simulink model "EHB_speedgoat_R2020a_V1"  (R2020a)
settings: Solver=FixedStepDiscrete  StartTime=0.0  StopTime=inf  FixedStep=0.001  RelTol=1e-3  EnableMultiTasking=on
model workspace (MAT data in the model file):
  A : Simulink.Signal (value not decoded)
  B : Simulink.Signal (value not decoded)
  C : Simulink.Signal (value not decoded)
  D : Simulink.Signal (value not decoded)
  E : Simulink.Signal (value not decoded)
  calin = [-9.96 -7.98 -5.98 -3.99 -1.994 0 1.995 3.992 5.99 7.98 9.97]
  calout = [-10 -8 -6 -4 -2 0 2 4 6 8 10]
symbols that are objects in the model workspace (value not decoded): C, D
undefined symbols (not defined in the file): Com1, none, ts_IO612
libraries: simulink x1436, xpcethercatlib x1223, yisutbxlib_utilities x256, xpcutilitieslib x156, hdlsllib x145, canmsglib x46, speedgoatlib_IO602_4 x11, speedgoatlib_IO611 x7, slrttcplib x4, CanManageLib x3, slrtlib x3, xpcseriallib x2
(part 7 of 30)

== system EHB_speedgoat_R2020a_V1/保留/TIF_02/CB3012_01/Res2Cmd6 ==
  ResVal : Inport
  Add : Sum  Inputs=-+
  Constant : Constant
  Divide : Product  Inputs=*/  OutDataTypeStr=uint16  RndMeth=Round
  MaxResVal : Constant  Value=1e6  OutDataTypeStr=Inherit: Inherit via back propagation
  Switch : Switch  Criteria=u2 > Threshold  OutDataTypeStr=Inherit: Inherit via back propagation
  zero : Constant  Value=0  OutDataTypeStr=Inherit: Inherit via back propagation
  CmdVal : Outport
  wires:
  MaxResVal/1 -> Divide/1
  Divide/1 -> Switch/1
  Switch/1 -> CmdVal/1
  zero/1 -> Switch/3
  ResVal/1 -> Add/2
  Add/1 -> Divide/2, Switch/2
  Constant/1 -> Add/1

== system EHB_speedgoat_R2020a_V1/保留/TIF_02/CB3012_01/Res2Cmd7 ==
  ResVal : Inport
  Add : Sum  Inputs=-+
  Constant : Constant
  Divide : Product  Inputs=*/  OutDataTypeStr=uint16  RndMeth=Round
  MaxResVal : Constant  Value=1e6  OutDataTypeStr=Inherit: Inherit via back propagation
  Switch : Switch  Criteria=u2 > Threshold  OutDataTypeStr=Inherit: Inherit via back propagation
  zero : Constant  Value=0  OutDataTypeStr=Inherit: Inherit via back propagation
  CmdVal : Outport
  wires:
  Constant/1 -> Add/1
  Add/1 -> Switch/2, Divide/2
  ResVal/1 -> Add/2
  zero/1 -> Switch/3
  Switch/1 -> CmdVal/1
  Divide/1 -> Switch/1
  MaxResVal/1 -> Divide/1

== system EHB_speedgoat_R2020a_V1/保留/TIF_02/CB3012_01/Res2Cmd8 ==
  ResVal : Inport
  Add : Sum  Inputs=-+
  Constant : Constant
  Divide : Product  Inputs=*/  OutDataTypeStr=uint16  RndMeth=Round
  MaxResVal : Constant  Value=1e6  OutDataTypeStr=Inherit: Inherit via back propagation
  Switch : Switch  Criteria=u2 > Threshold  OutDataTypeStr=Inherit: Inherit via back propagation
  zero : Constant  Value=0  OutDataTypeStr=Inherit: Inherit via back propagation
  CmdVal : Outport
  wires:
  MaxResVal/1 -> Divide/1
  Divide/1 -> Switch/1
  Switch/1 -> CmdVal/1
  zero/1 -> Switch/3
  ResVal/1 -> Add/2
  Add/1 -> Divide/2, Switch/2
  Constant/1 -> Add/1

== system EHB_speedgoat_R2020a_V1/保留/TIF_02/CB3012_01/Res2Cmd9 ==
  ResVal : Inport
  Add : Sum  Inputs=-+
  Constant : Constant
  Divide : Product  Inputs=*/  OutDataTypeStr=uint16  RndMeth=Round
  MaxResVal : Constant  Value=1e6  OutDataTypeStr=Inherit: Inherit via back propagation
  Switch : Switch  Criteria=u2 > Threshold  OutDataTypeStr=Inherit: Inherit via back propagation
  zero : Constant  Value=0  OutDataTypeStr=Inherit: Inherit via back propagation
  CmdVal : Outport
  wires:
  Constant/1 -> Add/1
  Add/1 -> Switch/2, Divide/2
  ResVal/1 -> Add/2
  zero/1 -> Switch/3
  Switch/1 -> CmdVal/1
  Divide/1 -> Switch/1
  MaxResVal/1 -> Divide/1

== system EHB_speedgoat_R2020a_V1/保留/TIF_03/CB1032_3/DIO ==
  DI : Subsystem  mask(simucat_di){deviceID=0, boxNum=Box 3 (Digital Board), channel1=on, channel2=on, channel3=on, channel4=on, channel5=on, channel6=on, channel7=on, channel8=on, channel9=on, channel10=on, channel11=on, channel12=on, channel13=on, channel14=on, channel15=on, channel16=on, channel17=on, channel18=on, channel19=on, channel20=on, channel21=on, channel22=on, channel23=on, channel24=on, channel25=on, channel26=on, channel27=on, channel28=on, channel29=on, channel30=on, channel31=on, channel32=on}
      mask prompts: deviceID "Device Index:"; boxNum "Select a box:"; channel1 "1"; channel2 "2"; channel3 "3"; channel4 "4"; channel5 "5"; channel6 "6"; channel7 "7"; channel8 "8"; channel9 "9"; channel10 "10"; channel11 "11"; channel12 "12"; channel13 "13"; channel14 "14"; channel15 "15"; channel16 "16"; channel17 "17"; channel18 "18"; channel19 "19"; channel20 "20"; channel21 "21"; channel22 "22"; channel23 "23"; channel24 "24"; channel25 "25"; channel26 "26"; channel27 "27"; channel28 "28"; channel29 "29"; channel30 "30"; channel31 "31"; channel32 "32"
      mask help:
      | SimuCat系列数字板卡驱动模块。
      | 功能：数字量输入。通道数：32
      mask TypeOptions deviceID: 0 | 1 | 2 | 3 | 4 | 5 | 6 | 7 | 8 | 9 | 10 | 11 | 12 | 13 | 14 | 15
      mask TypeOptions boxNum: Box 1 (Digital Board) | Box 2 (Digital Board) | Box 3 (Digital Board) | Box 4 (Digital Board)
      mask DialogControl refreshButton Prompt: Refresh
      mask DialogControl refreshButton Callback: ystbx.mask.callbacks.refreshBoxList
      mask DialogControl selectChannel Prompt: Select channels:
      mask DialogControl Dummy Prompt: (Add text here)
      mask DialogControl channelSelectAll Prompt: Select All
      mask DialogControl channelSelectAll Callback: ystbx.mask.callbacks.selectAllChannels();
      mask DialogControl channelClearAll Prompt: Clear All
      mask DialogControl channelClearAll Callback: ystbx.mask.callbacks.clearAllChannels();
      mask DialogControl applyButton Prompt: Apply Modification
      mask DialogControl applyButton Callback: ystbx.mask.callbacks.maskApply();
      mask Display: disp('CB1032(Digital Board)\ndigital signal input\nNetwork Device 0\nBox 3 (Digital Board)');port_label('output',1,'DI_CH1');port_label('output',2,'DI_CH2');port_label('output',3,'DI_CH3');port_label('output',4,'DI_CH4');port_label('output',5,'DI_CH5');port_label('output',6,'DI_CH6');port_label('output',7,'DI_CH7');port_label('output',8,'DI_CH8');port_label('output',9,'DI_CH9');port_label('output',10,'DI_CH10');port_label('output',11,'DI_CH11');port_label('output',12,'DI_CH12');port_label('output',13,'DI_CH13');port_label('output',14,'DI_CH14');port_label('output',15,'DI_CH15');port_label('output',16,'DI_CH16');port_label('output',17,'DI_CH17');port_label('output',18,'DI_CH18');port_label('output',19,'DI_CH19');port_label('output',20,'DI_CH20');port_label('output',21,'DI_CH21');port_label('output',22,'DI_CH22');port_label('output',23,'DI_CH23');port_label('output',24,'DI_CH24');port_label('output',25,'DI_CH25');port_label('output',26,'DI_CH26');port_label('output',27,'DI_CH27');port_label('output',28,'DI_CH28');port_label('output',29,'DI_CH29');port_label('output',30,'DI_CH30');port_label('output',31,'DI_CH31');port_label('output',32,'DI_CH32');
  DI_{1..32} (32 alike) : Gain  OutDataTypeStr=Inherit: Inherit via back propagation
  DO : Subsystem  mask(simucat_do){deviceID=0, boxNum=Box 3 (Digital Board), channel1=on, channel2=on, channel3=on, channel4=on, channel5=on, channel6=on, channel7=on, channel8=on, channel9=on, channel10=on, channel11=on, channel12=on, channel13=on, channel14=on, channel15=on, channel16=on, channel17=on, channel18=on, channel19=on, channel20=on, channel21=on, channel22=on, channel23=on, channel24=on, channel25=on, channel26=on, channel27=on, channel28=on, channel29=on, channel30=on, channel31=on, channel32=on, enableSetMode=off}
      mask prompts: deviceID "Device Index:"; boxNum "Select a box:"; channel1 "1"; channel2 "2"; channel3 "3"; channel4 "4"; channel5 "5"; channel6 "6"; channel7 "7"; channel8 "8"; channel9 "9"; channel10 "10"; channel11 "11"; channel12 "12"; channel13 "13"; channel14 "14"; channel15 "15"; channel16 "16"; channel17 "17"; channel18 "18"; channel19 "19"; channel20 "20"; channel21 "21"; channel22 "22"; channel23 "23"; channel24 "24"; channel25 "25"; channel26 "26"; channel27 "27"; channel28 "28"; channel29 "29"; channel30 "30"; channel31 "31"; channel32 "32"; enableSetMode "Enable SetMode"
      mask help:
      | SimuCat系列数字板卡驱动模块。
      | 功能：数字量输出。通道数：32
      mask TypeOptions deviceID: 0 | 1 | 2 | 3 | 4 | 5 | 6 | 7 | 8 | 9 | 10 | 11 | 12 | 13 | 14 | 15
      mask TypeOptions boxNum: Box 1 (Digital Board) | Box 2 (Digital Board) | Box 3 (Digital Board) | Box 4 (Digital Board)
      mask DialogControl refreshButton Prompt: Refresh
      mask DialogControl refreshButton Callback: ystbx.mask.callbacks.refreshBoxList
      mask DialogControl selectChannel Prompt: Select channels:
      mask DialogControl Dummy Prompt: (Add text here)
      mask DialogControl channelSelectAll Prompt: Select All
      mask DialogControl channelSelectAll Callback: ystbx.mask.callbacks.selectAllChannels();
      mask DialogControl channelClearAll Prompt: Clear All
      mask DialogControl channelClearAll Callback: ystbx.mask.callbacks.clearAllChannels();
      mask DialogControl applyButton Prompt: Apply Modification
      mask DialogControl applyButton Callback: ystbx.mask.callbacks.maskApply();
      mask Display: disp('CB1032(Digital Board)\ndigital signal output\nNetwork Device 0\nBox 3 (Digital Board)');port_label('input',1,'DO_CH1');port_label('input',2,'DO_CH2');port_label('input',3,'DO_CH3');port_label('input',4,'DO_CH4');port_label('input',5,'DO_CH5');port_label('input',6,'DO_CH6');port_label('input',7,'DO_CH7');port_label('input',8,'DO_CH8');port_label('input',9,'DO_CH9');port_label('input',10,'DO_CH10');port_label('input',11,'DO_CH11');port_label('input',12,'DO_CH12');port_label('input',13,'DO_CH13');port_label('input',14,'DO_CH14');port_label('input',15,'DO_CH15');port_label('input',16,'DO_CH16');port_label('input',17,'DO_CH17');port_label('input',18,'DO_CH18');port_label('input',19,'DO_CH19');port_label('input',20,'DO_CH20');port_label('input',21,'DO_CH21');port_label('input',22,'DO_CH22');port_label('input',23,'DO_CH23');port_label('input',24,'DO_CH24');port_label('input',25,'DO_CH25');port_label('input',26,'DO_CH26');port_label('input',27,'DO_CH27');port_label('input',28,'DO_CH28');port_label('input',29,'DO_CH29');port_label('input',30,'DO_CH30');port_label('input',31,'DO_CH31');port_label('input',32,'DO_CH32');
  DO_{1..32} (32 alike) : Constant  Value=0  OutDataTypeStr=Inherit: Inherit via back propagation
  Display{64..95} (32 alike) : Display
  wires:
  DI_28/1 -> Display85/1  "DI_28"
  DI_20/1 -> Display75/1  "DI_20"
  DI_7/1 -> Display68/1  "DI_7"
  DI_26/1 -> Display84/1  "DI_26"
  DI_12/1 -> Display81/1  "DI_12"
  DI_4/1 -> Display65/1  "DI_4"
  DI_18/1 -> Display82/1  "DI_18"
  DI_22/1 -> Display77/1  "DI_22"
  DI_25/1 -> Display80/1  "DI_25"
  DI_8/1 -> Display69/1  "DI_8"
  DI_11/1 -> Display72/1  "DI_11"
  DI_9/1 -> Display70/1  "DI_9"
  DI_1/1 -> Display64/1  "DI_1"
  DI_15/1 -> Display92/1  "DI_15"
  DI_3/1 -> Display95/1  "DI_3"
  DI_10/1 -> Display73/1  "DI_10"
  DI_5/1 -> Display66/1  "DI_5"
  DI_16/1 -> Display94/1  "DI_16"
  DI_2/1 -> Display71/1  "DI_2"
  DI_17/1 -> Display74/1  "DI_17"
  DI_14/1 -> Display91/1  "DI_14"
  DI_6/1 -> Display67/1  "DI_6"
  DI_13/1 -> Display93/1  "DI_13"
  DI_29/1 -> Display88/1  "DI_29"
  DI_19/1 -> Display90/1  "DI_19"
  DI_24/1 -> Display79/1  "DI_24"
  DI_30/1 -> Display86/1  "DI_30"
  DI_32/1 -> Display89/1  "DI_32"
  DI_27/1 -> Display83/1  "DI_27"
  DI_23/1 -> Display78/1  "DI_23"
  DI_31/1 -> Display87/1  "DI_31"
  DI_21/1 -> Display76/1  "DI_21"
  DO_1/1 -> DO/1(DO_CH1)  "DO_1"
  DO_2/1 -> DO/2(DO_CH2)  "DO_2"
  DO_3/1 -> DO/3(DO_CH3)  "DO_3"
  DO_4/1 -> DO/4(DO_CH4)  "DO_4"
  DO_5/1 -> DO/5(DO_CH5)  "DO_5"
  DO_6/1 -> DO/6(DO_CH6)  "DO_6"
  DO_7/1 -> DO/7(DO_CH7)  "DO_7"
  DO_8/1 -> DO/8(DO_CH8)  "DO_8"
  DO_9/1 -> DO/9(DO_CH9)  "DO_9"
  DO_10/1 -> DO/10(DO_CH10)  "DO_10"
  DO_11/1 -> DO/11(DO_CH11)  "DO_11"
  DO_12/1 -> DO/12(DO_CH12)  "DO_12"
  DO_13/1 -> DO/13(DO_CH13)  "DO_13"
  DO_14/1 -> DO/14(DO_CH14)  "DO_14"
  DO_15/1 -> DO/15(DO_CH15)  "DO_15"
  DO_16/1 -> DO/16(DO_CH16)  "DO_16"
  DO_17/1 -> DO/17(DO_CH17)  "DO_17"
  DO_18/1 -> DO/18(DO_CH18)  "DO_18"
  DO_19/1 -> DO/19(DO_CH19)  "DO_19"
  DO_20/1 -> DO/20(DO_CH20)  "DO_20"
  DO_21/1 -> DO/21(DO_CH21)  "DO_21"
  DO_22/1 -> DO/22(DO_CH22)  "DO_22"
  DO_23/1 -> DO/23(DO_CH23)  "DO_23"
  DO_24/1 -> DO/24(DO_CH24)  "DO_24"
  DO_25/1 -> DO/25(DO_CH25)  "DO_25"
  DO_26/1 -> DO/26(DO_CH26)  "DO_26"
  DO_27/1 -> DO/27(DO_CH27)  "DO_27"
  DO_28/1 -> DO/28(DO_CH28)  "DO_28"
  DO_29/1 -> DO/29(DO_CH29)  "DO_29"
  DO_30/1 -> DO/30(DO_CH30)  "DO_30"
  DO_31/1 -> DO/31(DO_CH31)  "DO_31"
  DO_32/1 -> DO/32(DO_CH32)  "DO_32"
  DI/1(DI_CH1) -> DI_1/1
  DI/2(DI_CH2) -> DI_2/1
  DI/3(DI_CH3) -> DI_3/1
  DI/4(DI_CH4) -> DI_4/1
  DI/5(DI_CH5) -> DI_5/1
  DI/6(DI_CH6) -> DI_6/1
  DI/7(DI_CH7) -> DI_7/1
  DI/8(DI_CH8) -> DI_8/1
  DI/9(DI_CH9) -> DI_9/1
  DI/10(DI_CH10) -> DI_10/1
  DI/11(DI_CH11) -> DI_11/1
  DI/12(DI_CH12) -> DI_12/1
  DI/13(DI_CH13) -> DI_13/1
  DI/14(DI_CH14) -> DI_14/1
  DI/15(DI_CH15) -> DI_15/1
  DI/16(DI_CH16) -> DI_16/1
  DI/17(DI_CH17) -> DI_17/1
  DI/18(DI_CH18) -> DI_18/1
  DI/19(DI_CH19) -> DI_19/1
  DI/20(DI_CH20) -> DI_20/1
  DI/21(DI_CH21) -> DI_21/1
  DI/22(DI_CH22) -> DI_22/1
  DI/23(DI_CH23) -> DI_23/1
  DI/24(DI_CH24) -> DI_24/1
  DI/25(DI_CH25) -> DI_25/1
  DI/26(DI_CH26) -> DI_26/1
  DI/27(DI_CH27) -> DI_27/1
  DI/28(DI_CH28) -> DI_28/1
  DI/29(DI_CH29) -> DI_29/1
  DI/30(DI_CH30) -> DI_30/1
  DI/31(DI_CH31) -> DI_31/1
  DI/32(DI_CH32) -> DI_32/1

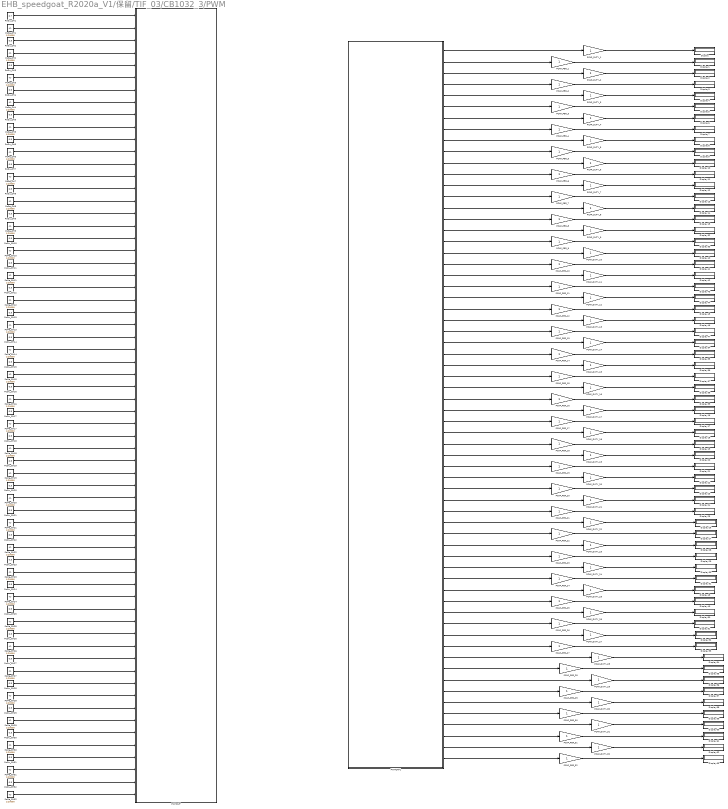
== system EHB_speedgoat_R2020a_V1/保留/TIF_03/CB1032_3/PWM ==
  Display{,1..63} (64 alike) : Display
  PCAP_DUTY_{1..32} (32 alike) : Gain
  PCAP_PER_{1..32} (32 alike) : Gain
  PWMCAP1 : Subsystem  mask(simucat_pwmcap){deviceID=0, boxNum=Box 3 (Digital Board), channel1=on, channel2=on, channel3=on, channel4=on, channel5=on, channel6=on, channel7=on, channel8=on, channel9=on, channel10=on, channel11=on, channel12=on, channel13=on, channel14=on, channel15=on, channel16=on, channel17=on, channel18=on, channel19=on, channel20=on, channel21=on, channel22=on, channel23=on, channel24=on, channel25=on, channel26=on, channel27=on, channel28=on, channel29=on, channel30=on, channel31=on, channel32=on, capMode=automatic}
      mask prompts: deviceID "Device Index:"; boxNum "Select a box:"; channel1 "1"; channel2 "2"; channel3 "3"; channel4 "4"; channel5 "5"; channel6 "6"; channel7 "7"; channel8 "8"; channel9 "9"; channel10 "10"; channel11 "11"; channel12 "12"; channel13 "13"; channel14 "14"; channel15 "15"; channel16 "16"; channel17 "17"; channel18 "18"; channel19 "19"; channel20 "20"; channel21 "21"; channel22 "22"; channel23 "23"; channel24 "24"; channel25 "25"; channel26 "26"; channel27 "27"; channel28 "28"; channel29 "29"; channel30 "30"; channel31 "31"; channel32 "32"; capMode "Cap Mode"
      mask help:
      | SimuCat系列数字板卡驱动模块。
      | 功能：PWM波捕获。通道数：32
      mask TypeOptions deviceID: 0 | 1 | 2 | 3 | 4 | 5 | 6 | 7 | 8 | 9 | 10 | 11 | 12 | 13 | 14 | 15
      mask TypeOptions boxNum: Box 1 (Digital Board) | Box 2 (Digital Board) | Box 3 (Digital Board) | Box 4 (Digital Board)
      mask TypeOptions capMode: automatic | manual
      mask DialogControl refreshButton Prompt: Refresh
      mask DialogControl refreshButton Callback: ystbx.mask.callbacks.refreshBoxList
      mask DialogControl selectChannel Prompt: Select channels:
      mask DialogControl Dummy Prompt: (Add text here)
      mask DialogControl channelSelectAll Prompt: Select All
      mask DialogControl channelSelectAll Callback: ystbx.mask.callbacks.selectAllChannels();
      mask DialogControl channelClearAll Prompt: Clear All
      mask DialogControl channelClearAll Callback: ystbx.mask.callbacks.clearAllChannels();
      mask DialogControl applyButton Prompt: Apply Modification
      mask DialogControl applyButton Callback: ystbx.mask.callbacks.maskApply();
      mask Display: disp('CB1032(Digital Board)\nPWM signal capture\nNetwork Device 0\nBox 3 (Digital Board)');port_label('output',1,'PWMCAP_DutyCycle_CH1');port_label('output',2,'PWMCAP_Period_CH1');port_label('output',3,'PWMCAP_DutyCycle_CH2');port_label('output',4,'PWMCAP_Period_CH2');port_label('output',5,'PWMCAP_DutyCycle_CH3');port_label('output',6,'PWMCAP_Period_CH3');port_label('output',7,'PWMCAP_DutyCycle_CH4');port_label('output',8,'PWMCAP_Period_CH4');port_label('output',9,'PWMCAP_DutyCycle_CH5');port_label('output',10,'PWMCAP_Period_CH5');port_label('output',11,'PWMCAP_DutyCycle_CH6');port_label('output',12,'PWMCAP_Period_CH6');port_label('output',13,'PWMCAP_DutyCycle_CH7');port_label('output',14,'PWMCAP_Period_CH7');port_label('output',15,'PWMCAP_DutyCycle_CH8');port_label('output',16,'PWMCAP_Period_CH8');port_label('output',17,'PWMCAP_DutyCycle_CH9');port_label('output',18,'PWMCAP_Period_CH9');port_label('output',19,'PWMCAP_DutyCycle_CH10');port_label('output',20,'PWMCAP_Period_CH10');port_label('output',21,'PWMCAP_DutyCycle_CH11');port_label('output',22,'PWMCAP_Period_CH11');port_label('output',23,'PWMCAP_DutyCycle_CH12');port_label('output',24,'PWMCAP_Period_CH12');port_label('output',25,'PWMCAP_DutyCycle_CH13');port_label('output',26,'PWMCAP_Period_CH13');port_label('output',27,'PWMCAP_DutyCycle_CH14');port_label('output',28,'PWMCAP_Period_CH14');port_label('output',29,'PWMCAP_DutyCycle_CH15');port_label('output',30,'PWMCAP_Period_CH15');port_label('output',31,'PWMCAP_DutyCycle_CH16');port_label('output',32,'PWMCAP_Period_CH16');port_label('output',33,'PWMCAP_DutyCycle_CH17');port_label('output',34,'PWMCAP_Period_CH17');port_label('output',35,'PWMCAP_DutyCycle_CH18');port_label('output',36,'PWMCAP_Period_CH18');port_label('output',37,'PWMCAP_DutyCycle_CH19');port_label('output',38,'PWMCAP_Period_CH19');port_label('output',39,'PWMCAP_DutyCycle_CH20');port_label('output',40,'PWMCAP_Period_CH20');port_label('output',41,'PWMCAP_DutyCycle_CH21');port_label('output',42,'PWMCAP_Period_CH21');port_label('output',43,'PWMCAP_DutyCycle_CH22');port_label('output',44,'PWMCAP_Period_CH22');port_label('output',45,'PWMCAP_DutyCycle_CH23');port_label('output',46,'PWMCAP_Period_CH23');port_label('output',47,'PWMCAP_DutyCycle_CH24');port_label('output',48,'PWMCAP_Period_CH24');port_label('output',49,'PWMCAP_DutyCycle_CH25');port_label('output',50,'PWMCAP_Period_CH25');port_label('output',51,'PWMCAP_DutyCycle_CH26');port_label('output',52,'PWMCAP_Period_CH26');port_label('output',53,'PWMCAP_DutyCycle_CH27');port_label('output',54,'PWMCAP_Period_CH27');port_label('output',55,'PWMCAP_DutyCycle_CH28');port_label('output',56,'PWMCAP_Period_CH28');port_label('output',57,'PWMCAP_DutyCycle_CH29');port_label('output',58,'PWMCAP_Period_CH29');port_label('output',59,'PWMCAP_DutyCycle_CH30');port_label('output',60,'PWMCAP_Period_CH30');port_label('output',61,'PWMCAP_DutyCycle_CH31');port_label('output',62,'PWMCAP_Period_CH31');port_label('output',63,'PWMCAP_DutyCycle_CH32');port_label('output',64,'PWMCAP_Period_CH32');
  PWMOUT : Subsystem  mask(simucat_pwmout){deviceID=0, boxNum=Box 3 (Digital Board), channel1=on, channel2=on, channel3=on, channel4=on, channel5=on, channel6=on, channel7=on, channel8=on, channel9=on, channel10=on, channel11=on, channel12=on, channel13=on, channel14=on, channel15=on, channel16=on, channel17=on, channel18=on, channel19=on, channel20=on, channel21=on, channel22=on, channel23=on, channel24=on, channel25=on, channel26=on, channel27=on, channel28=on, channel29=on, channel30=on, channel31=on, channel32=on}
      mask prompts: deviceID "Device Index:"; boxNum "Select a box:"; channel1 "1"; channel2 "2"; channel3 "3"; channel4 "4"; channel5 "5"; channel6 "6"; channel7 "7"; channel8 "8"; channel9 "9"; channel10 "10"; channel11 "11"; channel12 "12"; channel13 "13"; channel14 "14"; channel15 "15"; channel16 "16"; channel17 "17"; channel18 "18"; channel19 "19"; channel20 "20"; channel21 "21"; channel22 "22"; channel23 "23"; channel24 "24"; channel25 "25"; channel26 "26"; channel27 "27"; channel28 "28"; channel29 "29"; channel30 "30"; channel31 "31"; channel32 "32"
      mask help:
      | SimuCat系列数字板卡驱动模块。
      | 功能：PWM波输出。通道数：32
      mask TypeOptions deviceID: 0 | 1 | 2 | 3 | 4 | 5 | 6 | 7 | 8 | 9 | 10 | 11 | 12 | 13 | 14 | 15
      mask TypeOptions boxNum: Box 1 (Digital Board) | Box 2 (Digital Board) | Box 3 (Digital Board) | Box 4 (Digital Board)
      mask DialogControl refreshButton Prompt: Refresh
      mask DialogControl refreshButton Callback: ystbx.mask.callbacks.refreshBoxList
      mask DialogControl selectChannel Prompt: Select channels:
      mask DialogControl Dummy Prompt: (Add text here)
      mask DialogControl channelSelectAll Prompt: Select All
      mask DialogControl channelSelectAll Callback: ystbx.mask.callbacks.selectAllChannels();
      mask DialogControl channelClearAll Prompt: Clear All
      mask DialogControl channelClearAll Callback: ystbx.mask.callbacks.clearAllChannels();
      mask DialogControl applyButton Prompt: Apply Modification
      mask DialogControl applyButton Callback: ystbx.mask.callbacks.maskApply();
      mask Display: disp('CB1032(Digital Board)\nPWM signal output\nNetwork Device 0\nBox 3 (Digital Board)');port_label('input',1,'PWMOUT_DutyCycle_CH1');port_label('input',2,'PWMOUT_Period_CH1');port_label('input',3,'PWMOUT_DutyCycle_CH2');port_label('input',4,'PWMOUT_Period_CH2');port_label('input',5,'PWMOUT_DutyCycle_CH3');port_label('input',6,'PWMOUT_Period_CH3');port_label('input',7,'PWMOUT_DutyCycle_CH4');port_label('input',8,'PWMOUT_Period_CH4');port_label('input',9,'PWMOUT_DutyCycle_CH5');port_label('input',10,'PWMOUT_Period_CH5');port_label('input',11,'PWMOUT_DutyCycle_CH6');port_label('input',12,'PWMOUT_Period_CH6');port_label('input',13,'PWMOUT_DutyCycle_CH7');port_label('input',14,'PWMOUT_Period_CH7');port_label('input',15,'PWMOUT_DutyCycle_CH8');port_label('input',16,'PWMOUT_Period_CH8');port_label('input',17,'PWMOUT_DutyCycle_CH9');port_label('input',18,'PWMOUT_Period_CH9');port_label('input',19,'PWMOUT_DutyCycle_CH10');port_label('input',20,'PWMOUT_Period_CH10');port_label('input',21,'PWMOUT_DutyCycle_CH11');port_label('input',22,'PWMOUT_Period_CH11');port_label('input',23,'PWMOUT_DutyCycle_CH12');port_label('input',24,'PWMOUT_Period_CH12');port_label('input',25,'PWMOUT_DutyCycle_CH13');port_label('input',26,'PWMOUT_Period_CH13');port_label('input',27,'PWMOUT_DutyCycle_CH14');port_label('input',28,'PWMOUT_Period_CH14');port_label('input',29,'PWMOUT_DutyCycle_CH15');port_label('input',30,'PWMOUT_Period_CH15');port_label('input',31,'PWMOUT_DutyCycle_CH16');port_label('input',32,'PWMOUT_Period_CH16');port_label('input',33,'PWMOUT_DutyCycle_CH17');port_label('input',34,'PWMOUT_Period_CH17');port_label('input',35,'PWMOUT_DutyCycle_CH18');port_label('input',36,'PWMOUT_Period_CH18');port_label('input',37,'PWMOUT_DutyCycle_CH19');port_label('input',38,'PWMOUT_Period_CH19');port_label('input',39,'PWMOUT_DutyCycle_CH20');port_label('input',40,'PWMOUT_Period_CH20');port_label('input',41,'PWMOUT_DutyCycle_CH21');port_label('input',42,'PWMOUT_Period_CH21');port_label('input',43,'PWMOUT_DutyCycle_CH22');port_label('input',44,'PWMOUT_Period_CH22');port_label('input',45,'PWMOUT_DutyCycle_CH23');port_label('input',46,'PWMOUT_Period_CH23');port_label('input',47,'PWMOUT_DutyCycle_CH24');port_label('input',48,'PWMOUT_Period_CH24');port_label('input',49,'PWMOUT_DutyCycle_CH25');port_label('input',50,'PWMOUT_Period_CH25');port_label('input',51,'PWMOUT_DutyCycle_CH26');port_label('input',52,'PWMOUT_Period_CH26');port_label('input',53,'PWMOUT_DutyCycle_CH27');port_label('input',54,'PWMOUT_Period_CH27');port_label('input',55,'PWMOUT_DutyCycle_CH28');port_label('input',56,'PWMOUT_Period_CH28');port_label('input',57,'PWMOUT_DutyCycle_CH29');port_label('input',58,'PWMOUT_Period_CH29');port_label('input',59,'PWMOUT_DutyCycle_CH30');port_label('input',60,'PWMOUT_Period_CH30');port_label('input',61,'PWMOUT_DutyCycle_CH31');port_label('input',62,'PWMOUT_Period_CH31');port_label('input',63,'PWMOUT_DutyCycle_CH32');port_label('input',64,'PWMOUT_Period_CH32');
  PoDu_CH1 : Constant  Value=0.7
  PoDu_CH{2..32} (31 alike) : Constant  Value=0.5
  PoPe_CH{1..32} (32 alike) : Constant  Value=1/20000
  wires:
  PCAP_PER_27/1 -> Display53/1  "PCAP_PER_27"
  PCAP_PER_28/1 -> Display55/1  "PCAP_PER_28"
  PCAP_DUTY_8/1 -> Display14/1  "PCAP_DUTY_8"
  PCAP_DUTY_12/1 -> Display44/1  "PCAP_DUTY_12"
  PCAP_DUTY_9/1 -> Display32/1  "PCAP_DUTY_9"
  PCAP_PER_9/1 -> Display33/1  "PCAP_PER_9"
  PCAP_DUTY_20/1 -> Display22/1  "PCAP_DUTY_20"
  PCAP_PER_22/1 -> Display27/1  "PCAP_PER_22"
  PCAP_DUTY_4/1 -> Display6/1  "PCAP_DUTY_4"
  PCAP_PER_1/1 -> Display1/1  "PCAP_PER_1"
  PCAP_DUTY_5/1 -> Display8/1  "PCAP_DUTY_5"
  PCAP_DUTY_24/1 -> Display30/1  "PCAP_DUTY_24"
  PCAP_PER_10/1 -> Display41/1  "PCAP_PER_10"
  PCAP_PER_5/1 -> Display9/1  "PCAP_PER_5"
  PCAP_DUTY_23/1 -> Display28/1  "PCAP_DUTY_23"
  PCAP_PER_30/1 -> Display59/1  "PCAP_PER_30"
  PCAP_PER_23/1 -> Display29/1  "PCAP_PER_23"
  PCAP_DUTY_14/1 -> Display34/1  "PCAP_DUTY_14"
  PCAP_DUTY_22/1 -> Display26/1  "PCAP_DUTY_22"
  PCAP_PER_25/1 -> Display49/1  "PCAP_PER_25"
  PCAP_DUTY_13/1 -> Display46/1  "PCAP_DUTY_13"
  PCAP_DUTY_11/1 -> Display42/1  "PCAP_DUTY_11"
  PCAP_DUTY_31/1 -> Display60/1  "PCAP_DUTY_31"
  PCAP_PER_3/1 -> Display5/1  "PCAP_PER_3"
  PCAP_DUTY_29/1 -> Display56/1  "PCAP_DUTY_29"
  PCAP_DUTY_10/1 -> Display40/1  "PCAP_DUTY_10"
  PCAP_PER_14/1 -> Display35/1  "PCAP_PER_14"
  PCAP_PER_16/1 -> Display39/1  "PCAP_PER_16"
  PCAP_DUTY_30/1 -> Display58/1  "PCAP_DUTY_30"
  PCAP_DUTY_19/1 -> Display20/1  "PCAP_DUTY_19"
  PCAP_PER_31/1 -> Display61/1  "PCAP_PER_31"
  PCAP_PER_21/1 -> Display25/1  "PCAP_PER_21"
  PCAP_PER_20/1 -> Display23/1  "PCAP_PER_20"
  PCAP_DUTY_26/1 -> Display50/1  "PCAP_DUTY_26"
  PCAP_DUTY_7/1 -> Display12/1  "PCAP_DUTY_7"
  PCAP_PER_17/1 -> Display17/1  "PCAP_PER_17"
  PCAP_DUTY_25/1 -> Display48/1  "PCAP_DUTY_25"
  PCAP_PER_24/1 -> Display31/1  "PCAP_PER_24"
  PCAP_DUTY_18/1 -> Display18/1  "PCAP_DUTY_18"
  PCAP_PER_18/1 -> Display19/1  "PCAP_PER_18"
  PCAP_PER_32/1 -> Display63/1  "PCAP_PER_32"
  PCAP_DUTY_6/1 -> Display10/1  "PCAP_DUTY_6"
  PCAP_PER_8/1 -> Display15/1  "PCAP_PER_8"
  PCAP_DUTY_17/1 -> Display16/1  "PCAP_DUTY_17"
  PCAP_DUTY_15/1 -> Display36/1  "PCAP_DUTY_15"
  PCAP_DUTY_16/1 -> Display38/1  "PCAP_DUTY_16"
  PCAP_DUTY_21/1 -> Display24/1  "PCAP_DUTY_21"
  PCAP_DUTY_28/1 -> Display54/1  "PCAP_DUTY_28"
  PCAP_PER_11/1 -> Display43/1  "PCAP_PER_11"
  PCAP_PER_13/1 -> Display47/1  "PCAP_PER_13"
  PCAP_DUTY_2/1 -> Display2/1  "PCAP_DUTY_2"
  PCAP_PER_2/1 -> Display3/1  "PCAP_PER_2"
  PCAP_PER_19/1 -> Display21/1  "PCAP_PER_19"
  PCAP_PER_7/1 -> Display13/1  "PCAP_PER_7"
  PCAP_DUTY_27/1 -> Display52/1  "PCAP_DUTY_27"
  PCAP_PER_15/1 -> Display37/1  "PCAP_PER_15"
  PCAP_DUTY_32/1 -> Display62/1  "PCAP_DUTY_32"
  PCAP_PER_29/1 -> Display57/1  "PCAP_PER_29"
  PCAP_DUTY_1/1 -> Display/1  "PCAP_DUTY_1"
  PCAP_PER_6/1 -> Display11/1  "PCAP_PER_6"
  PCAP_DUTY_3/1 -> Display4/1  "PCAP_DUTY_3"
  PCAP_PER_26/1 -> Display51/1  "PCAP_PER_26"
  PCAP_PER_12/1 -> Display45/1  "PCAP_PER_12"
  PCAP_PER_4/1 -> Display7/1  "PCAP_PER_4"
  PoDu_CH1/1 -> PWMOUT/1(PWMOUT_DutyCycle_CH1)  "PoDu_CH17"
  PoPe_CH1/1 -> PWMOUT/2(PWMOUT_Period_CH1)  "PoPe_CH17"
  PoDu_CH2/1 -> PWMOUT/3(PWMOUT_DutyCycle_CH2)  "PoDu_CH18"
  PoPe_CH2/1 -> PWMOUT/4(PWMOUT_Period_CH2)  "PoPe_CH18"
  PoDu_CH3/1 -> PWMOUT/5(PWMOUT_DutyCycle_CH3)  "PoDu_CH19"
  PoPe_CH3/1 -> PWMOUT/6(PWMOUT_Period_CH3)  "PoPe_CH19"
  PoDu_CH4/1 -> PWMOUT/7(PWMOUT_DutyCycle_CH4)  "PoDu_CH20"
  PoPe_CH4/1 -> PWMOUT/8(PWMOUT_Period_CH4)  "PoPe_CH20"
  PoDu_CH5/1 -> PWMOUT/9(PWMOUT_DutyCycle_CH5)  "PoDu_CH21"
  PoPe_CH5/1 -> PWMOUT/10(PWMOUT_Period_CH5)  "PoPe_CH21"
  PoDu_CH6/1 -> PWMOUT/11(PWMOUT_DutyCycle_CH6)  "PoDu_CH22"
  PoPe_CH6/1 -> PWMOUT/12(PWMOUT_Period_CH6)  "PoPe_CH22"
  PoDu_CH7/1 -> PWMOUT/13(PWMOUT_DutyCycle_CH7)  "PoDu_CH23"
  PoPe_CH7/1 -> PWMOUT/14(PWMOUT_Period_CH7)  "PoPe_CH23"
  PoDu_CH8/1 -> PWMOUT/15(PWMOUT_DutyCycle_CH8)  "PoDu_CH24"
  PoPe_CH8/1 -> PWMOUT/16(PWMOUT_Period_CH8)  "PoPe_CH24"
  PoDu_CH9/1 -> PWMOUT/17(PWMOUT_DutyCycle_CH9)  "PoDu_CH25"
  PoPe_CH9/1 -> PWMOUT/18(PWMOUT_Period_CH9)  "PoPe_CH25"
  PoDu_CH10/1 -> PWMOUT/19(PWMOUT_DutyCycle_CH10)  "PoDu_CH26"
  PoPe_CH10/1 -> PWMOUT/20(PWMOUT_Period_CH10)  "PoPe_CH26"
  PoDu_CH11/1 -> PWMOUT/21(PWMOUT_DutyCycle_CH11)  "PoDu_CH27"
  PoPe_CH11/1 -> PWMOUT/22(PWMOUT_Period_CH11)  "PoPe_CH27"
  PoDu_CH12/1 -> PWMOUT/23(PWMOUT_DutyCycle_CH12)  "PoDu_CH28"
  PoPe_CH12/1 -> PWMOUT/24(PWMOUT_Period_CH12)  "PoPe_CH28"
  PoDu_CH13/1 -> PWMOUT/25(PWMOUT_DutyCycle_CH13)  "PoDu_CH29"
  PoPe_CH13/1 -> PWMOUT/26(PWMOUT_Period_CH13)  "PoPe_CH29"
  PoDu_CH14/1 -> PWMOUT/27(PWMOUT_DutyCycle_CH14)  "PoDu_CH30"
  PoPe_CH14/1 -> PWMOUT/28(PWMOUT_Period_CH14)  "PoPe_CH30"
  PoDu_CH15/1 -> PWMOUT/29(PWMOUT_DutyCycle_CH15)  "PoDu_CH31"
  PoPe_CH15/1 -> PWMOUT/30(PWMOUT_Period_CH15)  "PoPe_CH31"
  PoDu_CH16/1 -> PWMOUT/31(PWMOUT_DutyCycle_CH16)  "PoDu_CH32"
  PoPe_CH16/1 -> PWMOUT/32(PWMOUT_Period_CH16)  "PoPe_CH32"
  PoDu_CH17/1 -> PWMOUT/33(PWMOUT_DutyCycle_CH17)  "PoDu_CH17"
  PoPe_CH17/1 -> PWMOUT/34(PWMOUT_Period_CH17)  "PoPe_CH17"
  PoDu_CH18/1 -> PWMOUT/35(PWMOUT_DutyCycle_CH18)  "PoDu_CH18"
  PoPe_CH18/1 -> PWMOUT/36(PWMOUT_Period_CH18)  "PoPe_CH18"
  PoDu_CH19/1 -> PWMOUT/37(PWMOUT_DutyCycle_CH19)  "PoDu_CH19"
  PoPe_CH19/1 -> PWMOUT/38(PWMOUT_Period_CH19)  "PoPe_CH19"
  PoDu_CH20/1 -> PWMOUT/39(PWMOUT_DutyCycle_CH20)  "PoDu_CH20"
  PoPe_CH20/1 -> PWMOUT/40(PWMOUT_Period_CH20)  "PoPe_CH20"
  PoDu_CH21/1 -> PWMOUT/41(PWMOUT_DutyCycle_CH21)  "PoDu_CH21"
  PoPe_CH21/1 -> PWMOUT/42(PWMOUT_Period_CH21)  "PoPe_CH21"
  PoDu_CH22/1 -> PWMOUT/43(PWMOUT_DutyCycle_CH22)  "PoDu_CH22"
  PoPe_CH22/1 -> PWMOUT/44(PWMOUT_Period_CH22)  "PoPe_CH22"
  PoDu_CH23/1 -> PWMOUT/45(PWMOUT_DutyCycle_CH23)  "PoDu_CH23"
  PoPe_CH23/1 -> PWMOUT/46(PWMOUT_Period_CH23)  "PoPe_CH23"
  PoDu_CH24/1 -> PWMOUT/47(PWMOUT_DutyCycle_CH24)  "PoDu_CH24"
  PoPe_CH24/1 -> PWMOUT/48(PWMOUT_Period_CH24)  "PoPe_CH24"
  PoDu_CH25/1 -> PWMOUT/49(PWMOUT_DutyCycle_CH25)  "PoDu_CH25"
  PoPe_CH25/1 -> PWMOUT/50(PWMOUT_Period_CH25)  "PoPe_CH25"
  PoDu_CH26/1 -> PWMOUT/51(PWMOUT_DutyCycle_CH26)  "PoDu_CH26"
  PoPe_CH26/1 -> PWMOUT/52(PWMOUT_Period_CH26)  "PoPe_CH26"
  PoDu_CH27/1 -> PWMOUT/53(PWMOUT_DutyCycle_CH27)  "PoDu_CH27"
  PoPe_CH27/1 -> PWMOUT/54(PWMOUT_Period_CH27)  "PoPe_CH27"
  PoDu_CH28/1 -> PWMOUT/55(PWMOUT_DutyCycle_CH28)  "PoDu_CH28"
  PoPe_CH28/1 -> PWMOUT/56(PWMOUT_Period_CH28)  "PoPe_CH28"
  PoDu_CH29/1 -> PWMOUT/57(PWMOUT_DutyCycle_CH29)  "PoDu_CH29"
  PoPe_CH29/1 -> PWMOUT/58(PWMOUT_Period_CH29)  "PoPe_CH29"
  PoDu_CH30/1 -> PWMOUT/59(PWMOUT_DutyCycle_CH30)  "PoDu_CH30"
  PoPe_CH30/1 -> PWMOUT/60(PWMOUT_Period_CH30)  "PoPe_CH30"
  PoDu_CH31/1 -> PWMOUT/61(PWMOUT_DutyCycle_CH31)  "PoDu_CH31"
  PoPe_CH31/1 -> PWMOUT/62(PWMOUT_Period_CH31)  "PoPe_CH31"
  PoDu_CH32/1 -> PWMOUT/63(PWMOUT_DutyCycle_CH32)  "PoDu_CH32"
  PoPe_CH32/1 -> PWMOUT/64(PWMOUT_Period_CH32)  "PoPe_CH32"
  PWMCAP1/2(PWMCAP_Period_CH1) -> PCAP_PER_1/1
  PWMCAP1/4(PWMCAP_Period_CH2) -> PCAP_PER_2/1
  PWMCAP1/6(PWMCAP_Period_CH3) -> PCAP_PER_3/1
  PWMCAP1/8(PWMCAP_Period_CH4) -> PCAP_PER_4/1
  PWMCAP1/10(PWMCAP_Period_CH5) -> PCAP_PER_5/1
  PWMCAP1/12(PWMCAP_Period_CH6) -> PCAP_PER_6/1
  PWMCAP1/14(PWMCAP_Period_CH7) -> PCAP_PER_7/1
  PWMCAP1/16(PWMCAP_Period_CH8) -> PCAP_PER_8/1
  PWMCAP1/18(PWMCAP_Period_CH9) -> PCAP_PER_9/1
  PWMCAP1/20(PWMCAP_Period_CH10) -> PCAP_PER_10/1
  PWMCAP1/22(PWMCAP_Period_CH11) -> PCAP_PER_11/1
  PWMCAP1/24(PWMCAP_Period_CH12) -> PCAP_PER_12/1
  PWMCAP1/26(PWMCAP_Period_CH13) -> PCAP_PER_13/1
  PWMCAP1/28(PWMCAP_Period_CH14) -> PCAP_PER_14/1
  PWMCAP1/30(PWMCAP_Period_CH15) -> PCAP_PER_15/1
  PWMCAP1/32(PWMCAP_Period_CH16) -> PCAP_PER_16/1
  PWMCAP1/34(PWMCAP_Period_CH17) -> PCAP_PER_17/1
  PWMCAP1/36(PWMCAP_Period_CH18) -> PCAP_PER_18/1
  PWMCAP1/38(PWMCAP_Period_CH19) -> PCAP_PER_19/1
  PWMCAP1/40(PWMCAP_Period_CH20) -> PCAP_PER_20/1
  PWMCAP1/42(PWMCAP_Period_CH21) -> PCAP_PER_21/1
  PWMCAP1/44(PWMCAP_Period_CH22) -> PCAP_PER_22/1
  PWMCAP1/46(PWMCAP_Period_CH23) -> PCAP_PER_23/1
  PWMCAP1/48(PWMCAP_Period_CH24) -> PCAP_PER_24/1
  PWMCAP1/50(PWMCAP_Period_CH25) -> PCAP_PER_25/1
  PWMCAP1/52(PWMCAP_Period_CH26) -> PCAP_PER_26/1
  PWMCAP1/54(PWMCAP_Period_CH27) -> PCAP_PER_27/1
  PWMCAP1/56(PWMCAP_Period_CH28) -> PCAP_PER_28/1
  PWMCAP1/58(PWMCAP_Period_CH29) -> PCAP_PER_29/1
  PWMCAP1/60(PWMCAP_Period_CH30) -> PCAP_PER_30/1
  PWMCAP1/62(PWMCAP_Period_CH31) -> PCAP_PER_31/1
  PWMCAP1/64(PWMCAP_Period_CH32) -> PCAP_PER_32/1
  PWMCAP1/1(PWMCAP_DutyCycle_CH1) -> PCAP_DUTY_1/1
  PWMCAP1/3(PWMCAP_DutyCycle_CH2) -> PCAP_DUTY_2/1
  PWMCAP1/5(PWMCAP_DutyCycle_CH3) -> PCAP_DUTY_3/1
  PWMCAP1/7(PWMCAP_DutyCycle_CH4) -> PCAP_DUTY_4/1
  PWMCAP1/9(PWMCAP_DutyCycle_CH5) -> PCAP_DUTY_5/1
  PWMCAP1/11(PWMCAP_DutyCycle_CH6) -> PCAP_DUTY_6/1
  PWMCAP1/13(PWMCAP_DutyCycle_CH7) -> PCAP_DUTY_7/1
  PWMCAP1/15(PWMCAP_DutyCycle_CH8) -> PCAP_DUTY_8/1
  PWMCAP1/17(PWMCAP_DutyCycle_CH9) -> PCAP_DUTY_9/1
  PWMCAP1/19(PWMCAP_DutyCycle_CH10) -> PCAP_DUTY_10/1
  PWMCAP1/21(PWMCAP_DutyCycle_CH11) -> PCAP_DUTY_11/1
  PWMCAP1/23(PWMCAP_DutyCycle_CH12) -> PCAP_DUTY_12/1
  PWMCAP1/25(PWMCAP_DutyCycle_CH13) -> PCAP_DUTY_13/1
  PWMCAP1/27(PWMCAP_DutyCycle_CH14) -> PCAP_DUTY_14/1
  PWMCAP1/29(PWMCAP_DutyCycle_CH15) -> PCAP_DUTY_15/1
  PWMCAP1/31(PWMCAP_DutyCycle_CH16) -> PCAP_DUTY_16/1
  PWMCAP1/33(PWMCAP_DutyCycle_CH17) -> PCAP_DUTY_17/1
  PWMCAP1/35(PWMCAP_DutyCycle_CH18) -> PCAP_DUTY_18/1
  PWMCAP1/37(PWMCAP_DutyCycle_CH19) -> PCAP_DUTY_19/1
  PWMCAP1/39(PWMCAP_DutyCycle_CH20) -> PCAP_DUTY_20/1
  PWMCAP1/41(PWMCAP_DutyCycle_CH21) -> PCAP_DUTY_21/1
  PWMCAP1/43(PWMCAP_DutyCycle_CH22) -> PCAP_DUTY_22/1
  PWMCAP1/45(PWMCAP_DutyCycle_CH23) -> PCAP_DUTY_23/1
  PWMCAP1/47(PWMCAP_DutyCycle_CH24) -> PCAP_DUTY_24/1
  PWMCAP1/49(PWMCAP_DutyCycle_CH25) -> PCAP_DUTY_25/1
  PWMCAP1/51(PWMCAP_DutyCycle_CH26) -> PCAP_DUTY_26/1
  PWMCAP1/53(PWMCAP_DutyCycle_CH27) -> PCAP_DUTY_27/1
  PWMCAP1/55(PWMCAP_DutyCycle_CH28) -> PCAP_DUTY_28/1
  PWMCAP1/57(PWMCAP_DutyCycle_CH29) -> PCAP_DUTY_29/1
  PWMCAP1/59(PWMCAP_DutyCycle_CH30) -> PCAP_DUTY_30/1
  PWMCAP1/61(PWMCAP_DutyCycle_CH31) -> PCAP_DUTY_31/1
  PWMCAP1/63(PWMCAP_DutyCycle_CH32) -> PCAP_DUTY_32/1

== system EHB_speedgoat_R2020a_V1/保留/TIF_03/CB1032_4/DIO ==
  DI : Subsystem  mask(simucat_di){deviceID=0, boxNum=Box 4 (Digital Board), channel1=on, channel2=on, channel3=on, channel4=on, channel5=on, channel6=on, channel7=on, channel8=on, channel9=on, channel10=on, channel11=on, channel12=on, channel13=on, channel14=on, channel15=on, channel16=on, channel17=on, channel18=on, channel19=on, channel20=on, channel21=on, channel22=on, channel23=on, channel24=on, channel25=on, channel26=on, channel27=on, channel28=on, channel29=on, channel30=on, channel31=on, channel32=on}
      mask prompts: deviceID "Device Index:"; boxNum "Select a box:"; channel1 "1"; channel2 "2"; channel3 "3"; channel4 "4"; channel5 "5"; channel6 "6"; channel7 "7"; channel8 "8"; channel9 "9"; channel10 "10"; channel11 "11"; channel12 "12"; channel13 "13"; channel14 "14"; channel15 "15"; channel16 "16"; channel17 "17"; channel18 "18"; channel19 "19"; channel20 "20"; channel21 "21"; channel22 "22"; channel23 "23"; channel24 "24"; channel25 "25"; channel26 "26"; channel27 "27"; channel28 "28"; channel29 "29"; channel30 "30"; channel31 "31"; channel32 "32"
      mask help:
      | SimuCat系列数字板卡驱动模块。
      | 功能：数字量输入。通道数：32
      mask TypeOptions deviceID: 0 | 1 | 2 | 3 | 4 | 5 | 6 | 7 | 8 | 9 | 10 | 11 | 12 | 13 | 14 | 15
      mask TypeOptions boxNum: Box 1 (Digital Board) | Box 2 (Digital Board) | Box 3 (Digital Board) | Box 4 (Digital Board)
      mask DialogControl refreshButton Prompt: Refresh
      mask DialogControl refreshButton Callback: ystbx.mask.callbacks.refreshBoxList
      mask DialogControl selectChannel Prompt: Select channels:
      mask DialogControl Dummy Prompt: (Add text here)
      mask DialogControl channelSelectAll Prompt: Select All
      mask DialogControl channelSelectAll Callback: ystbx.mask.callbacks.selectAllChannels();
      mask DialogControl channelClearAll Prompt: Clear All
      mask DialogControl channelClearAll Callback: ystbx.mask.callbacks.clearAllChannels();
      mask DialogControl applyButton Prompt: Apply Modification
      mask DialogControl applyButton Callback: ystbx.mask.callbacks.maskApply();
      mask Display: disp('CB1032(Digital Board)\ndigital signal input\nNetwork Device 0\nBox 4 (Digital Board)');port_label('output',1,'DI_CH1');port_label('output',2,'DI_CH2');port_label('output',3,'DI_CH3');port_label('output',4,'DI_CH4');port_label('output',5,'DI_CH5');port_label('output',6,'DI_CH6');port_label('output',7,'DI_CH7');port_label('output',8,'DI_CH8');port_label('output',9,'DI_CH9');port_label('output',10,'DI_CH10');port_label('output',11,'DI_CH11');port_label('output',12,'DI_CH12');port_label('output',13,'DI_CH13');port_label('output',14,'DI_CH14');port_label('output',15,'DI_CH15');port_label('output',16,'DI_CH16');port_label('output',17,'DI_CH17');port_label('output',18,'DI_CH18');port_label('output',19,'DI_CH19');port_label('output',20,'DI_CH20');port_label('output',21,'DI_CH21');port_label('output',22,'DI_CH22');port_label('output',23,'DI_CH23');port_label('output',24,'DI_CH24');port_label('output',25,'DI_CH25');port_label('output',26,'DI_CH26');port_label('output',27,'DI_CH27');port_label('output',28,'DI_CH28');port_label('output',29,'DI_CH29');port_label('output',30,'DI_CH30');port_label('output',31,'DI_CH31');port_label('output',32,'DI_CH32');
  DI_{1..32} (32 alike) : Gain  OutDataTypeStr=Inherit: Inherit via back propagation
  DO : Subsystem  mask(simucat_do){deviceID=0, boxNum=Box 4 (Digital Board), channel1=on, channel2=on, channel3=on, channel4=on, channel5=on, channel6=on, channel7=on, channel8=on, channel9=on, channel10=on, channel11=on, channel12=on, channel13=on, channel14=on, channel15=on, channel16=on, channel17=on, channel18=on, channel19=on, channel20=on, channel21=on, channel22=on, channel23=on, channel24=on, channel25=on, channel26=on, channel27=on, channel28=on, channel29=on, channel30=on, channel31=on, channel32=on, enableSetMode=off}
      mask prompts: deviceID "Device Index:"; boxNum "Select a box:"; channel1 "1"; channel2 "2"; channel3 "3"; channel4 "4"; channel5 "5"; channel6 "6"; channel7 "7"; channel8 "8"; channel9 "9"; channel10 "10"; channel11 "11"; channel12 "12"; channel13 "13"; channel14 "14"; channel15 "15"; channel16 "16"; channel17 "17"; channel18 "18"; channel19 "19"; channel20 "20"; channel21 "21"; channel22 "22"; channel23 "23"; channel24 "24"; channel25 "25"; channel26 "26"; channel27 "27"; channel28 "28"; channel29 "29"; channel30 "30"; channel31 "31"; channel32 "32"; enableSetMode "Enable SetMode"
      mask help:
      | SimuCat系列数字板卡驱动模块。
      | 功能：数字量输出。通道数：32
      mask TypeOptions deviceID: 0 | 1 | 2 | 3 | 4 | 5 | 6 | 7 | 8 | 9 | 10 | 11 | 12 | 13 | 14 | 15
      mask TypeOptions boxNum: Box 1 (Digital Board) | Box 2 (Digital Board) | Box 3 (Digital Board) | Box 4 (Digital Board)
      mask DialogControl refreshButton Prompt: Refresh
      mask DialogControl refreshButton Callback: ystbx.mask.callbacks.refreshBoxList
      mask DialogControl selectChannel Prompt: Select channels:
      mask DialogControl Dummy Prompt: (Add text here)
      mask DialogControl channelSelectAll Prompt: Select All
      mask DialogControl channelSelectAll Callback: ystbx.mask.callbacks.selectAllChannels();
      mask DialogControl channelClearAll Prompt: Clear All
      mask DialogControl channelClearAll Callback: ystbx.mask.callbacks.clearAllChannels();
      mask DialogControl applyButton Prompt: Apply Modification
      mask DialogControl applyButton Callback: ystbx.mask.callbacks.maskApply();
      mask Display: disp('CB1032(Digital Board)\ndigital signal output\nNetwork Device 0\nBox 4 (Digital Board)');port_label('input',1,'DO_CH1');port_label('input',2,'DO_CH2');port_label('input',3,'DO_CH3');port_label('input',4,'DO_CH4');port_label('input',5,'DO_CH5');port_label('input',6,'DO_CH6');port_label('input',7,'DO_CH7');port_label('input',8,'DO_CH8');port_label('input',9,'DO_CH9');port_label('input',10,'DO_CH10');port_label('input',11,'DO_CH11');port_label('input',12,'DO_CH12');port_label('input',13,'DO_CH13');port_label('input',14,'DO_CH14');port_label('input',15,'DO_CH15');port_label('input',16,'DO_CH16');port_label('input',17,'DO_CH17');port_label('input',18,'DO_CH18');port_label('input',19,'DO_CH19');port_label('input',20,'DO_CH20');port_label('input',21,'DO_CH21');port_label('input',22,'DO_CH22');port_label('input',23,'DO_CH23');port_label('input',24,'DO_CH24');port_label('input',25,'DO_CH25');port_label('input',26,'DO_CH26');port_label('input',27,'DO_CH27');port_label('input',28,'DO_CH28');port_label('input',29,'DO_CH29');port_label('input',30,'DO_CH30');port_label('input',31,'DO_CH31');port_label('input',32,'DO_CH32');
  DO_{1..31} (31 alike) : Constant  Value=0  OutDataTypeStr=Inherit: Inherit via back propagation
  DO_32 : Constant  OutDataTypeStr=Inherit: Inherit via back propagation
  Display{64..95} (32 alike) : Display
  wires:
  DI_1/1 -> Display64/1  "DI_1"
  DI_7/1 -> Display68/1  "DI_7"
  DI_31/1 -> Display87/1  "DI_31"
  DI_21/1 -> Display76/1  "DI_21"
  DI_9/1 -> Display70/1  "DI_9"
  DI_27/1 -> Display83/1  "DI_27"
  DI_11/1 -> Display72/1  "DI_11"
  DI_28/1 -> Display85/1  "DI_28"
  DI_6/1 -> Display67/1  "DI_6"
  DI_14/1 -> Display91/1  "DI_14"
  DI_24/1 -> Display79/1  "DI_24"
  DI_30/1 -> Display86/1  "DI_30"
  DI_8/1 -> Display69/1  "DI_8"
  DI_5/1 -> Display66/1  "DI_5"
  DI_32/1 -> Display89/1  "DI_32"
  DI_3/1 -> Display95/1  "DI_3"
  DI_22/1 -> Display77/1  "DI_22"
  DI_17/1 -> Display74/1  "DI_17"
  DI_20/1 -> Display75/1  "DI_20"
  DI_2/1 -> Display71/1  "DI_2"
  DI_23/1 -> Display78/1  "DI_23"
  DI_19/1 -> Display90/1  "DI_19"
  DI_10/1 -> Display73/1  "DI_10"
  DI_25/1 -> Display80/1  "DI_25"
  DI_16/1 -> Display94/1  "DI_16"
  DI_26/1 -> Display84/1  "DI_26"
  DI_13/1 -> Display93/1  "DI_13"
  DI_4/1 -> Display65/1  "DI_4"
  DI_18/1 -> Display82/1  "DI_18"
  DI_12/1 -> Display81/1  "DI_12"
  DI_15/1 -> Display92/1  "DI_15"
  DI_29/1 -> Display88/1  "DI_29"
  DO_1/1 -> DO/1(DO_CH1)  "DO_1"
  DO_2/1 -> DO/2(DO_CH2)  "DO_2"
  DO_3/1 -> DO/3(DO_CH3)  "DO_3"
  DO_4/1 -> DO/4(DO_CH4)  "DO_4"
  DO_5/1 -> DO/5(DO_CH5)  "DO_5"
  DO_6/1 -> DO/6(DO_CH6)  "DO_6"
  DO_7/1 -> DO/7(DO_CH7)  "DO_7"
  DO_8/1 -> DO/8(DO_CH8)  "DO_8"
  DO_9/1 -> DO/9(DO_CH9)  "DO_9"
  DO_10/1 -> DO/10(DO_CH10)  "DO_10"
  DO_11/1 -> DO/11(DO_CH11)  "DO_11"
  DO_12/1 -> DO/12(DO_CH12)  "DO_12"
  DO_13/1 -> DO/13(DO_CH13)  "DO_13"
  DO_14/1 -> DO/14(DO_CH14)  "DO_14"
  DO_15/1 -> DO/15(DO_CH15)  "DO_15"
  DO_16/1 -> DO/16(DO_CH16)  "DO_16"
  DO_17/1 -> DO/17(DO_CH17)  "DO_17"
  DO_18/1 -> DO/18(DO_CH18)  "DO_18"
  DO_19/1 -> DO/19(DO_CH19)  "DO_19"
  DO_20/1 -> DO/20(DO_CH20)  "DO_20"
  DO_21/1 -> DO/21(DO_CH21)  "DO_21"
  DO_22/1 -> DO/22(DO_CH22)  "DO_22"
  DO_23/1 -> DO/23(DO_CH23)  "DO_23"
  DO_24/1 -> DO/24(DO_CH24)  "DO_24"
  DO_25/1 -> DO/25(DO_CH25)  "DO_25"
  DO_26/1 -> DO/26(DO_CH26)  "DO_26"
  DO_27/1 -> DO/27(DO_CH27)  "DO_27"
  DO_28/1 -> DO/28(DO_CH28)  "DO_28"
  DO_29/1 -> DO/29(DO_CH29)  "DO_29"
  DO_30/1 -> DO/30(DO_CH30)  "DO_30"
  DO_31/1 -> DO/31(DO_CH31)  "DO_31"
  DO_32/1 -> DO/32(DO_CH32)  "DO_32"
  DI/1(DI_CH1) -> DI_1/1
  DI/2(DI_CH2) -> DI_2/1
  DI/3(DI_CH3) -> DI_3/1
  DI/4(DI_CH4) -> DI_4/1
  DI/5(DI_CH5) -> DI_5/1
  DI/6(DI_CH6) -> DI_6/1
  DI/7(DI_CH7) -> DI_7/1
  DI/8(DI_CH8) -> DI_8/1
  DI/9(DI_CH9) -> DI_9/1
  DI/10(DI_CH10) -> DI_10/1
  DI/11(DI_CH11) -> DI_11/1
  DI/12(DI_CH12) -> DI_12/1
  DI/13(DI_CH13) -> DI_13/1
  DI/14(DI_CH14) -> DI_14/1
  DI/15(DI_CH15) -> DI_15/1
  DI/16(DI_CH16) -> DI_16/1
  DI/17(DI_CH17) -> DI_17/1
  DI/18(DI_CH18) -> DI_18/1
  DI/19(DI_CH19) -> DI_19/1
  DI/20(DI_CH20) -> DI_20/1
  DI/21(DI_CH21) -> DI_21/1
  DI/22(DI_CH22) -> DI_22/1
  DI/23(DI_CH23) -> DI_23/1
  DI/24(DI_CH24) -> DI_24/1
  DI/25(DI_CH25) -> DI_25/1
  DI/26(DI_CH26) -> DI_26/1
  DI/27(DI_CH27) -> DI_27/1
  DI/28(DI_CH28) -> DI_28/1
  DI/29(DI_CH29) -> DI_29/1
  DI/30(DI_CH30) -> DI_30/1
  DI/31(DI_CH31) -> DI_31/1
  DI/32(DI_CH32) -> DI_32/1
